simulink model "Simulink_Model"  (R2022b)
settings: Solver=VariableStepAuto  StartTime=0.0  StopTime=10  RelTol=1e-3
settings Model: Creator=Admin  LastModifiedBy=Admin

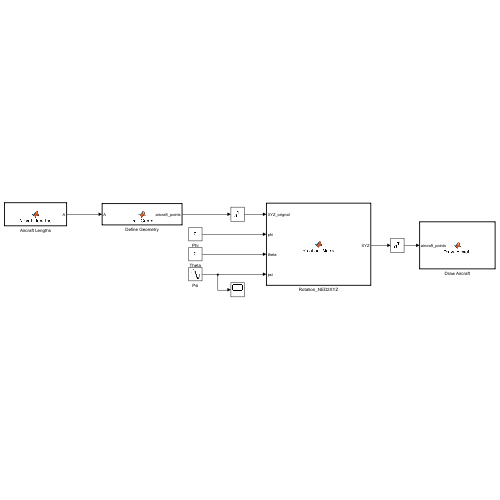
[thumbnail: Simulink's stored preview of the top-level diagram]
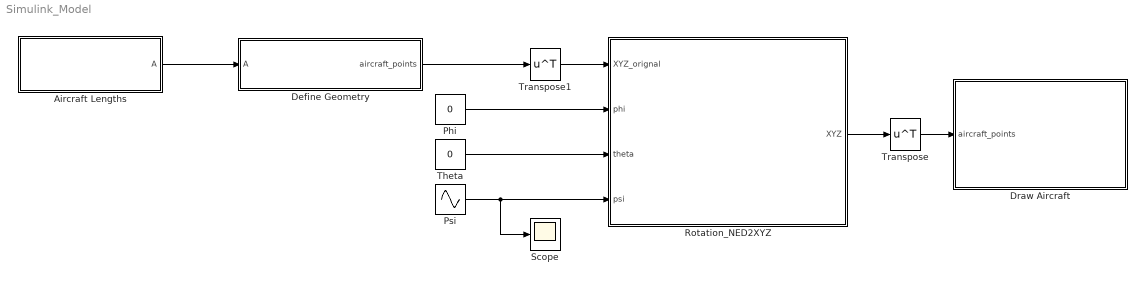
== system Simulink_Model ==
  Aircraft Lengths : MATLAB Function  TreatAsAtomicUnit=on
  Define Geometry : MATLAB Function  TreatAsAtomicUnit=on
  Draw Aircraft : MATLAB Function  TreatAsAtomicUnit=on
  Phi : Constant  Value=0
  Psi : Sin  Amplitude=45  SampleTime=1
  Rotation_NED2XYZ : MATLAB Function  TreatAsAtomicUnit=on
  Scope : Scope
  Theta : Constant  Value=0
  Transpose : Math  Operator=transpose
  Transpose1 : Math  Operator=transpose
  wires:
  Define Geometry/1(aircraft_points) -> Transpose1/1
  Phi/1 -> Rotation_NED2XYZ/2(phi)
  Theta/1 -> Rotation_NED2XYZ/3(theta)
  Aircraft Lengths/1(A) -> Define Geometry/1(A)
  Rotation_NED2XYZ/1(XYZ) -> Transpose/1
  Transpose/1 -> Draw Aircraft/1(aircraft_points)
  Transpose1/1 -> Rotation_NED2XYZ/1(XYZ_orignal)
  Psi/1 -> Scope/1, Rotation_NED2XYZ/4(psi)

== matlab function Simulink_Model/Rotation_NED2XYZ ==
  data: XYZ_orignal input; XYZ output; phi input; theta input; psi input
function XYZ = Rotation_Matrix(XYZ_orignal, phi, theta, psi)
R_roll = [1 0 0;
          0 cosd(phi) sind(phi);
          0 -sind(phi) cosd(phi);];

R_pitch = [cosd(theta) 0 -sind(theta);
           0 1 0;
           sind(theta) 0 cosd(theta);];

R_yaw = [cosd(psi) sind(psi) 0;
         -sind(psi) cosd(psi) 0;
         0 0 1;];

R = R_roll*R_pitch*R_yaw;
XYZ = (R*XYZ_orignal);
% set_angles(phi,theta,psi);
end

== matlab function Simulink_Model/Define Geometry ==
  data: A input; aircraft_points output
function aircraft_points= Def_Geom(A)
%%
% A(1), A(2), A(3), A(4), A(5), A(6), A(7), A(8), A(9), A(10), A(11)
% Matrix A is defined as the order of Aircraft part lengths as given above
% in order of appearnace. A is 11 X 1 Matrix
%%
% Geometry Variables
aircraft_points = [
            A(9), 0, 0; % Point 1
            A(10), A(7)/2, -A(8)/2; % Point 2
            A(10), -A(7)/2, -A(8)/2; % Point 3
            A(10), -A(7)/2, A(8)/2; % Point 4
            A(10), A(7)/2, A(8)/2; % Point 5
            -A(11), 0, 0; % Point 6
            0, A(2)/2, 0; % Point 7
            -A(1), A(2)/2, 0; % Point 8
            -A(1), -A(2)/2, 0; % Point 9
            0, -A(2)/2, 0; % Point 10
            -A(11)+A(3), A(4)/2,0; % Point 11
            -A(11), A(4)/2,0; % Point 12
            -A(11), -A(4)/2,0; % Point 13
            -A(11)+A(3), -A(4)/2,0; % Point 14
            -A(11)+A(6), 0, 0; % Point 15
            -A(11), 0, -A(5); % Point 16
            ];
end

== matlab function Simulink_Model/Aircraft Lengths ==
  data: A output
function A = Aircraft_lengths()
aircraft_lengths = [2 20 1 6 1.5 1.5 1.5 1.5 4 2 15];
A = aircraft_lengths;
end

== matlab function Simulink_Model/Draw Aircraft ==
  data: aircraft_points input
function Draw_Aircraft(aircraft_points)
aircraft_faces3 = [
            1 2 3; % Nose
            1 2 5; % Nose
            1 4 5; % Nose
            1 3 4; % Nose
            2 3 6; % Fuselage
            3 4 6; % Fuselage
            4 5 6; % Fuselage
            2 5 6; % Fuselage
            15 16 6; % Vertical Tail
            ];
aircraft_faces4 = [
            7 8 9 10; % Wing
            11 12 13 14; % Horizontal Tail
            2 3 4 5; % Nose-Fuselage
            ];
hold on
patch('Faces', aircraft_faces3,'Vertices', aircraft_points,'FaceColor', 'red')
patch('Faces', aircraft_faces4,'Vertices', aircraft_points,'FaceColor', 'blue')
xlabel("X-Label")
ylabel("Y-Label")
zlabel("Z-Label")
set(gca,"ZDir",'reverse')
axis equal
grid on
end
